simulink model "Clutchless_P2_Parallel_ETE"  (R2017b)
settings: Solver=FixedStepAuto  StartTime=0.0  StopTime=length(Speed)  FixedStep=0.01  MaxStep=0.01  RelTol=1e-3  EnableMultiTasking=on
PostLoadFcn:
  | , if any(exist('dsrtsu_mdlpostloadfcn', 'file') == [2, 3, 6]), try dsrtsu_mdlpostloadfcn('Execute', bdroot); catch fprintf('Error in PostLoadFcn (dsrtsu_mdlpostloadfcn) for model "%s":\n %s\n', bdroot, lasterr); end, end,
undefined symbols (not defined in the file): ABSEnable, Actuators, air, APP1_OOR, APP2_OOR, APP_Mismatch, Brk_Flt, cal, ClutchEngag, Clutchless_HSC_ETE, CS_On_Control, Driver, eng, Engine, EngOverTemp, ENGTRQ_MSMCH_Degraded_CP, ENGTRQ_MSMCH_ErrCritical_CP, ENGTRQ_MSMCH_LimpHome_CP, EngTrqMismatch, env, ess, ESSOverTemp, gb, KeyPos_Flt, KeyPosition, lib_Actuators, lib_Clutchless_HSC_ETE, lib_Driver, lib_EMachine_2017a, lib_Sensors_2017a, LossCAN, Machine, max_vehicle_rad_air_flow, MCUOverTemp, mot, MotDirMismatch, MotOverTemp, MotTrqMismatch, mph2ms, PRNDL_Flt, RegenBrkDisable, RegenFault, Sensors, ShiftLeverPosition, Speed, SW_CS_ON, SW_Engine_ON, t_amb, time, tloop
libraries: simulink x97, Pneumatic_lib x11, nesl_utility x9, EC2_libraries x7, powerlib_meascontrol x2, CalculationGallon x1, lib_Chassis x1, lib_DCDC x1, lib_Differential x1, lib_HVESS x1, fl_lib x1, lib_OBC x1
(part 3 of 9)

== system Clutchless_P2_Parallel_ETE/Camaro Plant Model/ICE Simple1/Engine Plant Modified/ECU Sensors ==
  In1 : Inport
  In2 : Inport  Port=2
  In3 : Inport  Port=3
  In4 : Inport  Port=4
  In5 : Inport  Port=5
  In6 : Inport  Port=6
  In7 : Inport  Port=7
  In8 : Inport  Port=8
  In9 : Inport  Port=9
  In10 : Inport  Port=10
  Bus Creator : BusCreator  Inputs=10
  Memory : Memory
  Out1 : Outport
  wires:
  In9/1 -> Bus Creator/9  "NOx_g/s"
  In1/1 -> Bus Creator/1  "EngActStdyStTorq_Nm"
  In2/1 -> Bus Creator/2  "EngSpd_RPM"
  In3/1 -> Bus Creator/3  "EngFuelFlow_g/s"
  In4/1 -> Bus Creator/4  "FuelLevelPct"
  In5/1 -> Bus Creator/5  "PE_0_1"
  In6/1 -> Bus Creator/6  "HC_g/s"
  In7/1 -> Bus Creator/7  "CO_g/s"
  Bus Creator/1 -> Memory/1
  In8/1 -> Bus Creator/8  "CO2_g/s"
  In10/1 -> Bus Creator/10  "Eng_Temp"
  Memory/1 -> Out1/1

== system Clutchless_P2_Parallel_ETE/Camaro Plant Model/ICE Simple1/Engine Plant Modified/Fuel Supply ==
  0 to 100 : Saturate
  Fuel Pump Disable : Constant  Value=0
  Fuel Volumn : Constant  Value=Engine.Fuel.Initial_Volumn
  Integrator : Integrator  LimitOutput=on  UpperSaturationLimit=Engine.FuelTank.Volume  LowerSaturationLimit=0
  L to % : Gain  Gain=100/Engine.FuelTank.Volume
  Sum : Sum  Inputs=+-
  Switch : Switch  Threshold=1
  g to L : Gain  Gain=1/Engine.Fuel.Density/1000
  Available Fuel : Outport
  tag scope: FuelLevelPct=global
  wires:
  0 to 100/1 -> [FuelLevelPct]
  L to %/1 -> 0 to 100/1
  Fuel Pump Disable/1 -> Switch/3
  g to L/1 -> Switch/1
  Integrator/1 -> g to L/1
  [AdvFuelFlowEst] -> Integrator/1
  [FuelPumpEnable] -> Switch/2
  Sum/1 -> L to %/1, Available Fuel/1
  Switch/1 -> Sum/2
  Fuel Volumn/1 -> Sum/1

== system Clutchless_P2_Parallel_ETE/Camaro Plant Model/ICE Simple1/Engine Plant Modified/Radiator ==
  note: Calculation of max air flow:
      |
      | The air flow reach the max in the scenario that only fan rejects all the heat coolant brings in
      |
      | The regular max CFM of a vehicle radiator fan is about 2000
      |
      | CFM=1.76* Q/delta T_air
      |
      | Where Q is the max amount of heat from coolant, assume that the max temperature drop of coolant
      | through radiator is 10 deg C
      |
      | Q= Mc_coolant* Cp_coolant* delta T_coolant=3500*0.26*10=9100w
      |
      | delta T_air=1.76*Q/CFM=1.76*9100/2000=8 degC
      |
      | Max Mc_air=Q/(Cp_air*delta T_air)=9100/(1006*8)=1.13 kg/s
  EngCltTmp : Inport
  Fans : Inport  Port=2
  " " : Product  Inputs=**
  " " : Gain  Gain=0.05
  Ambient Temp : Constant  Value=env.init.T_ambiant
  Compare To Zero : simulink/Logic and Bit Operations/Compare To Zero  relop===  OutDataTypeStr=uint8
  Constant : Constant
  Cp of Air : Constant  Value=air.init.specific_heat
  Cp of Air1 : Constant  Value=air.init.specific_heat
  Data Type Conversion1 : DataTypeConversion
  Divide by Zero Fix : Subsystem
  "Eng Mc=Q/(Cp*delta T) " : Product  Inputs=*/
  Q=Mc_air*Cp_air*delta T : Product  Inputs=***
  Saturation : Saturate  UpperLimit=max_vehicle_rad_air_flow  LowerLimit=-1
  Sum3 : Sum  Inputs=|-+
  Sum4 : Sum
  Sum5 : Sum  Inputs=|+-
  Switch : Switch  Threshold=1
  Terminator : Terminator
  vehspdflow : Gain  Gain=0.01
  tag scope: AirFlowRequest=global, Heat_Reject_Eng=global
  wires:
  Data Type Conversion1/1 -> " "/1
  Cp of Air1/1 -> Q=Mc_air*Cp_air*delta T/3
  Switch/1 -> Q=Mc_air*Cp_air*delta T/2  "eng act air flow in kg/s"
  Q=Mc_air*Cp_air*delta T/1 -> " "/2  "J/s"
  " "/1 -> [Heat_Reject_Eng]  "J"
  Saturation/1 -> Sum3/1  "Actual air flow"
  Sum3/1 -> Compare To Zero/1
  Compare To Zero/1 -> Switch/2  "request meet"
  Cp of Air/1 -> "Eng Mc=Q/(Cp*delta T) "/2  "Cp J/kg*C"
  Ambient Temp/1 -> Sum5/2  "25 deg C"
  Sum5/1 -> Divide by Zero Fix/2(Divide), Q=Mc_air*Cp_air*delta T/1  "Delta T = Tcoolant - Tambient"
  EngCltTmp/1 -> Sum5/1  "EngCltTmp in deg C"
  "Eng Mc=Q/(Cp*delta T) "/1 -> Switch/1, Sum3/2, [AirFlowRequest]  "Eng requested air flow in Kg/s"
  Sum4/1 -> Switch/3, Saturation/1  "Air Flow Recieved"
  Fans/1 -> Data Type Conversion1/1
  [VehSpdAvgDrvn_Eng] -> vehspdflow/1
  vehspdflow/1 -> Sum4/2
  [Heat_Transfer_Eng] -> Divide by Zero Fix/1(Multiply)  "heat generation in w"
  Divide by Zero Fix/1(Output) -> "Eng Mc=Q/(Cp*delta T) "/1
  " "/1 -> Sum4/1
  Constant/1 -> " "/1
  [AirFlowRequest] -> Terminator/1

== system Clutchless_P2_Parallel_ETE/Camaro Plant Model/ICE Simple1/Engine Plant Modified/Subsystem ==
  EngFuelFlow_g/s : Inport
  Eng_Temp : Inport  Port=2
  Rate Transition1 : RateTransition  OutPortSampleTime=1
  Rate Transition7 : RateTransition  OutPortSampleTime=1
  To Workspace2 : ToWorkspace  VariableName=EngCltTmp  SampleTime=-1
  To Workspace3 : ToWorkspace  VariableName=InstFuelConsmpRate  SampleTime=-1
  g/s 2 l/hr : Gain  Gain=0.001/0.7871*3600
  wires:
  EngFuelFlow_g/s/1 -> g/s 2 l/hr/1
  Eng_Temp/1 -> Rate Transition1/1
  Rate Transition1/1 -> To Workspace2/1
  g/s 2 l/hr/1 -> Rate Transition7/1
  Rate Transition7/1 -> To Workspace3/1

== system Clutchless_P2_Parallel_ETE/Camaro Plant Model/ICE Simple1/Inputs/Analog ==
  Out1 : Outport
  wires:
  [Analog] -> Out1/1

== system Clutchless_P2_Parallel_ETE/Camaro Plant Model/ICE Simple1/Inputs/CAN_from_HCU ==
  Bus Creator : BusCreator  Inputs=2
  Out1 : Outport
  wires:
  [HCU_to_EBCAN] -> Bus Creator/1
  [HCU_to_VEH_CAN] -> Bus Creator/2
  Bus Creator/1 -> Out1/1

== system Clutchless_P2_Parallel_ETE/Camaro Plant Model/ICE Simple1/Soft ECM/ECM_RollingAliveCnt ==
  Constant : Constant
  Constant1 : Constant  Value=0
  Rolling Alive Counter : Stateflow chart  TreatAsAtomicUnit=on
  Switch : Switch  Criteria=u2 > Threshold
  Out1 : Outport
  tag scope: ECM_CAN_fault=global
  wires:
  [ECM_CAN_fault] -> Switch/2
  Constant/1 -> Switch/1
  Rolling Alive Counter/1(RollingAliveCnt) -> Switch/3
  Switch/1 -> Out1/1  "ECM_RollingAliveCnt"
  Constant1/1 -> [ECM_CAN_fault]

== system Clutchless_P2_Parallel_ETE/Camaro Plant Model/ICE Simple1/Soft ECM/Fuel Consumption ==
  note: Total Fuel Consumed
  Fuel Consumption : Inport
  " " : Constant  Value=3600
  " tloop" : Constant  Value=0.01
  1/fuel density : Gain  Gain=1/Engine.Fuel.Density
  Add : Sum  Inputs=|++
  Add1 : Sum  Inputs=|++
  Constant3 : Constant  Value=Engine.Fuel.Lower_Heating_Value/1000
  Divide : Product  Inputs=*/
  Divide by Zero Fix : Subsystem
  Divide by Zero Fix1 : Subsystem
  Gain1 : Gain  Gain=0.001
  Memory : Memory
  Memory1 : Memory
  Product : Product  RndMeth=Zero
  Product1 : Product  RndMeth=Zero
  Product3 : Product  RndMeth=Zero
  Scope : Scope
  To Workspace1 : ToWorkspace  VariableName=eng_fuel_consump_mpl  SampleTime=-1
      settings: Decimation=WORKSPACE_DECIMATION
  To Workspace5 : ToWorkspace  VariableName=eng_wh_per_mile_hist  SampleTime=-1
      settings: Decimation=WORKSPACE_DECIMATION
  fuel consumption : Outport
  wires:
  Divide by Zero Fix1/1(Output) -> To Workspace5/1
  Divide/1 -> Add1/1  "Wh"
  Memory1/1 -> Add1/2
  Add1/1 -> Divide by Zero Fix1/2(Multiply), Memory1/1  "cumulative"
  Product/1 -> Product3/2  "W"
  Constant3/1 -> Product/2
  Divide by Zero Fix/1(Output) -> fuel consumption/1, To Workspace1/1, Scope/1
  [veh_dist_miles] -> Divide by Zero Fix1/1(Divide), Divide by Zero Fix/2(Multiply)  "miles"
  Product1/1 -> Add/1  "liter"
  1/fuel density/1 -> Product1/1  "liter/sec"
  Fuel Consumption/1 -> Product/1, Gain1/1  "g/s"
  Memory/1 -> Add/2
  Add/1 -> Divide by Zero Fix/1(Divide), Memory/1  "cumulative_liter"
  " tloop"/1 -> Product3/1, Product1/2
  Product3/1 -> Divide/1
  " "/1 -> Divide/2
  Gain1/1 -> 1/fuel density/1

== system Clutchless_P2_Parallel_ETE/Camaro Plant Model/ICE Simple1/Soft ECM/Logic/APP2TP ==
  APP : Inport
  EngSpd : Inport  Port=2
  f : TriggerPort  TriggerType=function-call  VariantControl=Variant
      settings: CopyFcn=Stateflow.SLINSF.SimulinkMan.removeBlockPreDeleteFcn  PreDeleteFcn=Stateflow.SLINSF.SimulinkMan.unsafePredeleteFcn
  Based on APP to TP test data from 2013 Malibu1 : Lookup_n-D  NumberOfTableDimensions=1  BreakpointsForDimension1=[0,1,2,3,4,5,6,7,8,9,10,11,12,13,14,15,16,17,18,19,20,21,22,23,24,25,26,27,28,29,30,31,32,33,34,35,36,37,38,39,40,41,42,43,44,45,46,48,51,55,60,66,100]  Table=[0,6.3,12.7686537241448,12.6326703204763,12.8888951657611,13.4307541011932,14.1739282202018,15.0532596030224,16.0198646102832,17.0384547356068,18.0848650172271,19.1437900086214,20.206727308158,21.2701286477589,22.3337585405773,23.3992604876916,24.4689307438132,25.5446996420107,26.6273204774486,27.7157659501418,28.8068321667249,29.8949502012373,30.9722052149229,32.0285631350456,33.0523048927199,34.0306682197568,34.9506970045247,35.8002982068255,36.5695063317874,37.2519554627699,37.846558853288,38.359396077948,38.8058077424007,39.2126977523099,39.6210431413345,40.0886114581279,40.6928857123509,41.5341968797017,42.7390639659588,44.4637416300428,46.8979753660875,50.2689642445339,54.8455312122302,60.9425009515619,68.9252852985734,79.2146762201353,81.9427,84.6943,87.2166,89.5096,91.3439,92.6051,100]  ExtrapMethod=Clip  UseLastTableValue=on  InternalRulePriority=Speed  RndMeth=Simplest  InputSameDT=on
  Based on APP to TP test data from 2013 Malibu2 : Lookup_n-D  Commented=on  NumberOfTableDimensions=1  BreakpointsForDimension1=[0,1,2,3,4,5,6,7,8,9,10,11,12,13,14,15,16,17,18,19,20,21,22,23,24,25,26,27,28,29,30,31,32,33,34,35,36,37,38,39,40,41,42,43,44,45,46,48,51,55,60,66,100]  Table=[0,7,12.5,16,16.5,17,18,19,21,23,25,28,29,30,32,35,37,39,41,44,47,48,48.6,49,50,51.5,52,53,53.25,53.5,55,56.75,57,58,60,64,68,72,73,74,75,76,77,77.5,78,80,82,85,87,89.5,91.5,93,100]  ExtrapMethod=Clip  UseLastTableValue=on  InternalRulePriority=Speed  RndMeth=Simplest  InputSameDT=on
  Display : Display
  Product : Product
  RPM Derating : Lookup_n-D  NumberOfTableDimensions=1  BreakpointsForDimension1=[0 1000 2000 3000 4000 5000 6000 7000]  Table=[1 1 1 1 1 1 1 0]  ExtrapMethod=Clip  UseLastTableValue=on  InternalRulePriority=Speed  RndMeth=Simplest  InputSameDT=on
  Saturation : Saturate  UpperLimit=100  LowerLimit=0
  TP : Outport
  wires:
  Product/1 -> TP/1
  EngSpd/1 -> RPM Derating/1
  RPM Derating/1 -> Product/2  "2"
  APP/1 -> Based on APP to TP test data from 2013 Malibu1/1, Display/1  "3"
  Based on APP to TP test data from 2013 Malibu1/1 -> Saturation/1  "1"
  Saturation/1 -> Product/1

== system Clutchless_P2_Parallel_ETE/Camaro Plant Model/Scopes/AxlTrq_to_EngTrq2/Ratio Filter ==
  Ratio : Inport
  Abs : Abs
  Compare To Zero : simulink/Logic and Bit Operations/Compare To Zero  relop===  OutDataTypeStr=boolean
  Constant : Constant  Value=cal.Time.TrnsOvrllEstTrqRatioSwitch
  Mature_Delay : EC2_libraries/Mature_Delay
      settings: SourceProductName=The database C:\Users\vrajm\AppData\Roaming\MathWorks\MATLAB\R2017b\slblocks_master.db is locked, or a table in the database is locked. (database is locked)
  Memory1 : Memory  InitialCondition=1
  Switch1 : Switch  Threshold=1
  Switch2 : Switch  Threshold=1
  Filtered_Ratio : Outport
  wires:
  Ratio/1 -> Compare To Zero/1, Abs/1
  Compare To Zero/1 -> Mature_Delay/1, Switch2/2
  Abs/1 -> Switch1/1, Switch2/3
  Switch1/1 -> Switch2/1
  Constant/1 -> Mature_Delay/2
  Mature_Delay/1 -> Switch1/2
  Memory1/1 -> Switch1/3
  Switch2/1 -> Filtered_Ratio/1, Memory1/1  "gear_ratio"

== system Clutchless_P2_Parallel_ETE/Camaro Plant Model/Scopes/AxlTrq_to_MtrTrq2/Ratio Filter ==
  Ratio : Inport
  Abs : Abs
  Compare To Zero : simulink/Logic and Bit Operations/Compare To Zero  relop===  OutDataTypeStr=boolean
  Constant : Constant  Value=cal.Time.TrnsOvrllEstTrqRatioSwitch
  Mature_Delay : EC2_libraries/Mature_Delay
      settings: SourceProductName=The database C:\Users\vrajm\AppData\Roaming\MathWorks\MATLAB\R2017b\slblocks_master.db is locked, or a table in the database is locked. (database is locked)
  Memory1 : Memory  InitialCondition=1
  Switch1 : Switch  Threshold=1
  Switch2 : Switch  Threshold=1
  Filtered_Ratio : Outport
  wires:
  Ratio/1 -> Compare To Zero/1, Abs/1
  Compare To Zero/1 -> Mature_Delay/1, Switch2/2
  Abs/1 -> Switch1/1, Switch2/3
  Switch1/1 -> Switch2/1
  Constant/1 -> Mature_Delay/2
  Mature_Delay/1 -> Switch1/2
  Memory1/1 -> Switch1/3
  Switch2/1 -> Filtered_Ratio/1, Memory1/1  "gear_ratio"

== system Clutchless_P2_Parallel_ETE/Clutchless_HSC_ETE/HSC/Camaro Fault Detection/Component Diagnostic ==
  note: Component Status Setting Rule
      | xxx_CompStatus could be 0, 1, 2 or 3
      | 0: component needs to be offline
      | 1: component needs torque plant to deliver creep torque
      | 2: component needs torque plant to limit maximum torque delivery
      | 3: component needs torque plant to operate normally
  note: Component Diagnostics
  SignalDiag : Inport
  Bus Creator : BusCreator  Inputs=6
  Driver Input Diagnostic : Subsystem
  ESS Component Diagnostic : Subsystem
  Engine Component Diagnostic : Subsystem
  Override Driver Status : Subsystem
  Override ESS Status : Subsystem
  Override Engine Status : Subsystem
  Override TCM Status : Subsystem
  Transmission Component Diagnostic : Subsystem
  CompDiag : Outport
  wires:
  SignalDiag/1 -> Engine Component Diagnostic/1(In1), Transmission Component Diagnostic/1(In1), Bus Creator/6, ESS Component Diagnostic/1(In1), Driver Input Diagnostic/1(In1)  "RawSig"
  Bus Creator/1 -> CompDiag/1
  Driver Input Diagnostic/1(Out1) -> Override Driver Status/1(In1)  "Diver_CompDiag"
  ESS Component Diagnostic/1(Out1) -> Override ESS Status/1(In1)  "ESS_CompDiag"
  Engine Component Diagnostic/1(Out1) -> Override Engine Status/1(In1)  "ECM_CompDiag"
  Transmission Component Diagnostic/1(Out1) -> Override TCM Status/1(In1)  "TCM_CompDiag"
  Override ESS Status/1(Out1) -> Bus Creator/2  "BMS_Status"
  Override Engine Status/1(Out1) -> Bus Creator/3  "ECM_Status"
  Override TCM Status/1(Out1) -> Bus Creator/5  "TCM_Status"
  Override Driver Status/1(Out1) -> Bus Creator/1  "Driver_Input_Status"
  Engine Component Diagnostic/2(Out2) -> Bus Creator/4  "EngTrqMismchType"

== system Clutchless_P2_Parallel_ETE/Clutchless_HSC_ETE/HSC/Camaro Fault Detection/Input Conversions ==
  note: Input Conversions and Override Switches
  note: These subsystems convert variable types to match those used in the
      | supervisor. In addition, override switches installed on each signal can
      | be used to manually override and signal for testing purposes
  RawSig : Inport
  BMS_Conversions : Subsystem
  Bus Creator : BusCreator  Inputs=5
  DriverInput_Conversions : Subsystem
  ECM_Conversions : Subsystem
  TCM_Conversions : Subsystem
  VehSig : Outport
  wires:
  DriverInput_Conversions/1(Out1) -> Bus Creator/1
  Bus Creator/1 -> VehSig/1  "InputConvAndOvrd"
  BMS_Conversions/1(Out1) -> Bus Creator/2
  RawSig/1 -> DriverInput_Conversions/1(In1), Bus Creator/5, TCM_Conversions/1(In1), ECM_Conversions/1(In1), BMS_Conversions/1(In1)  "RawSig"
  ECM_Conversions/1(Out1) -> Bus Creator/3
  TCM_Conversions/1(Out1) -> Bus Creator/4

== system Clutchless_P2_Parallel_ETE/Clutchless_HSC_ETE/HSC/Camaro Fault Detection/Signal Diagnostic ==
  note: These subsystems evaluate each signal for proper value range and other checks
  note: Signal Diagnostics
  VehSig : Inport
  Bus Creator : BusCreator  Inputs=5
  Driver Signal Diagnostic : Subsystem
  ESS Signal Diagnostic : Subsystem
  Engine Signal Diagnostic : Subsystem
  Subsystem1 : Subsystem
      mask Display: fprintf('Signal Naming Rule')
  Transmission Signal Diagnostic : Subsystem
  SignalDiag : Outport
  wires:
  VehSig/1 -> ESS Signal Diagnostic/1(Sensors1), Driver Signal Diagnostic/1(Sensors1), Engine Signal Diagnostic/1(Sensors1), Bus Creator/5, Transmission Signal Diagnostic/1(Sensors1)
  Driver Signal Diagnostic/1(Driver_SigDiag) -> Bus Creator/1  "Driver_SigDiag"
  ESS Signal Diagnostic/1(ESS_SigDiag) -> Bus Creator/2  "ESS_SigDiag"
  Engine Signal Diagnostic/1(Engine_SigDiag) -> Bus Creator/3  "Engine_SigDiag"
  Transmission Signal Diagnostic/1(Out2) -> Bus Creator/4  "Transmission_SigDiag"
  Bus Creator/1 -> SignalDiag/1  "SignalDiag"

== system Clutchless_P2_Parallel_ETE/Clutchless_HSC_ETE/HSC/Driver_Requests/APP_BPP to DrvIntndAxlTrq2 ==
  note: $Author: fy6949 $
      | $Rev: 577 $
      | $Date: 2017-1-19 08:53:15 -0500  $
  note: Note:Driver requested Axle Torque Calculation
  Sensors : Inport
  Diag : Inport  Port=2
  Controls : Inport  Port=3
  Bus Selector : BusSelector  OutputSignals=from_Analog.Driver_APP1,from_CAN.fromVEH_CAN.from_BCM.BrkPdlPos,from_CAN.fromEBCAN.from_ECM.VehSpdAvgDrvn,from_CAN.fromVEH_CAN.from_TCM.TrnGrRat,from_CAN.fromHV_CAN.from_MCU.INV_VCU_01.INV_Speed
  Bus Selector1 : BusSelector  OutputSignals=CompSig.RawSig.Driver_SigDiag.Drv_APP_Agree
  Bus Selector2 : BusSelector  OutputSignals=mode
  Post Driver Intnded Axle Torque : Subsystem
  Terminator : Terminator
  Terminator1 : Terminator
  IntndAxlTrq : Outport
  wires:
  Bus Selector2/1 -> Post Driver Intnded Axle Torque/5(Mode)  "<mode>"
  Bus Selector1/1 -> Terminator1/1  "<Drv_APP_Agree>"
  Diag/1 -> Bus Selector1/1
  Post Driver Intnded Axle Torque/2(BrkIntndAxlTrq) -> Terminator/1
  Bus Selector/1 -> Post Driver Intnded Axle Torque/1(APP)  "<Driver_APP1>"
  Bus Selector/4 -> Post Driver Intnded Axle Torque/4(TransGearRatio)  "<TrnGrRat>"
  Bus Selector/5 -> Post Driver Intnded Axle Torque/6(Motor_Speed)  "<INV_Speed>"
  Bus Selector/3 -> Post Driver Intnded Axle Torque/3(VehicleSpeed)  "<VehSpdAvgDrvn>"
  Bus Selector/2 -> Post Driver Intnded Axle Torque/2(BPP)  "<BrkPdlPos>"
  Post Driver Intnded Axle Torque/1(IntndAxlTrq) -> IntndAxlTrq/1
  Controls/1 -> Bus Selector2/1
  Sensors/1 -> Bus Selector/1

== system Clutchless_P2_Parallel_ETE/Clutchless_HSC_ETE/HSC/Powertrain Manager/HV Manager1 ==
  Sensors : Inport
  Controls : Inport  Port=2
  Axiomatic_Output_Manager : Subsystem
  BMS_Manager : Subsystem
  Bus Creator1 : BusCreator  Inputs=4
  DCDC Manager : Subsystem
  Inverter Manager : Subsystem
  OBC_Manager : Subsystem
  BMS_CAN : Outport
  HV_BUS_Status : Outport  Port=2
  OBC_CAN : Outport  Port=3
  OBC_Digital : Outport  Port=4
  BMS_Digital : Outport  Port=5
  Axiomatic_CAN : Outport  Port=6
  tag scope: MCU_CAN=global
  wires:
  [MCU_Status] -> BMS_Manager/3(In1)
  DCDC Manager/1(Out1) -> Bus Creator1/4
  Inverter Manager/3(MCU_Relay) -> Bus Creator1/3  "MCU_Relay"
  Axiomatic_Output_Manager/1(Axiomatic_CAN) -> Axiomatic_CAN/1
  BMS_Manager/3(BMS Digital) -> BMS_Digital/1
  BMS_Manager/1(BMS CAN) -> BMS_CAN/1
  Controls/1 -> Inverter Manager/3(Control), DCDC Manager/3(In2), DCDC Manager/2(In1), BMS_Manager/2(Controls)
  OBC_Manager/2(OBC_Digital) -> OBC_Digital/1
  OBC_Manager/1(OBC CAN) -> OBC_CAN/1
  [HV_BUS_Status] -> OBC_Manager/1(HV_Status)
  BMS_Manager/2(HV_BUS_Status) -> HV_BUS_Status/1, [HV_BUS_Status]  "HV_BUS_Status"
  [HV_BUS_Status] -> Axiomatic_Output_Manager/2(HV_Bus_Status)
  [HV_BUS_Status] -> Inverter Manager/1(HV_Bus_Status)  "HV_BUS_Status"
  Sensors/1 -> Inverter Manager/2(Sensors), OBC_Manager/2(Sensors), Axiomatic_Output_Manager/1(Sensors), DCDC Manager/1(BMSInput), BMS_Manager/1(Sensors)
  Inverter Manager/1(MCU_Status) -> Bus Creator1/1, [MCU_Status]  "MCU_Status"
  Inverter Manager/2(MCU_CAN) -> Bus Creator1/2  "MCU_CAN"
  Bus Creator1/1 -> [MCU_CAN]

== system Clutchless_P2_Parallel_ETE/Clutchless_HSC_ETE/HSC/Powertrain Manager/Output Conversion ==
  In1 : Inport
  In2 : Inport  Port=2
  In3 : Inport  Port=3
  In4 : Inport  Port=4
  In5 : Inport  Port=5
  In8 : Inport  Port=6
  In9 : Inport  Port=7
  In10 : Inport  Port=8
  In11 : Inport  Port=9
  Bus Creator : BusCreator  Inputs=14
  Bus Creator1 : BusCreator  Inputs=9
  Bus Selector2 : BusSelector  OutputSignals=powerMode,EnablePrplsn,ClutchEngage,EngAppReq,EngOnReq,MtrTrqCmd,EnableInverter,EngTrqCmd,HV_req,SysPwrMd_0_3,TransShftLvrPos,VehSpdAvgDrvn_kph,AccPos_Perc,SportsModeEnable
  Data Type Conversion{,2..3,5..13} (12 alike) : DataTypeConversion
  Memory : Memory
  Out1 : Outport
  wires:
  Bus Selector2/14 -> Bus Creator/14  "<SportsModeEnable>"
  In11/1 -> Bus Creator1/9
  In4/1 -> Bus Selector2/1
  Bus Selector2/1 -> Memory/1  "<powerMode>"
  Bus Selector2/2 -> Data Type Conversion2/1  "<EnablePrplsn>"
  Bus Selector2/3 -> Data Type Conversion3/1  "<ClutchEngage>"
  Bus Selector2/5 -> Data Type Conversion5/1  "<EngOnReq>"
  Bus Selector2/6 -> Data Type Conversion6/1  "<MtrTrqCmd>"
  Bus Selector2/7 -> Data Type Conversion7/1  "<EnableInverter>"
  Bus Selector2/8 -> Data Type Conversion8/1  "<EngTrqCmd>"
  Bus Selector2/9 -> Data Type Conversion9/1  "<HV_req>"
  Bus Selector2/10 -> Data Type Conversion10/1  "<SysPwrMd_0_3>"
  Data Type Conversion2/1 -> Bus Creator/2  "EnablePrplsn"
  Data Type Conversion3/1 -> Bus Creator/3  "ClutchEngage"
  Bus Selector2/4 -> Bus Creator/4  "<EngAppReq>"
  Data Type Conversion6/1 -> Bus Creator/6  "Torque_Command"
  Data Type Conversion7/1 -> Bus Creator/7  "Inverter_Enable"
  Data Type Conversion8/1 -> Bus Creator/8  "EngTrqCmd"
  Data Type Conversion9/1 -> Bus Creator/9  "HV_req"
  Data Type Conversion10/1 -> Bus Creator/10  "SysPwrMd"
  Data Type Conversion/1 -> Bus Creator/1  "powerMode"
  Data Type Conversion5/1 -> Bus Creator/5  "EngOnReq"
  Bus Creator1/1 -> Out1/1
  In1/1 -> Bus Creator1/1
  In2/1 -> Bus Creator1/2
  In3/1 -> Bus Creator1/3
  Bus Creator/1 -> Bus Creator1/4  "Controls"
  In5/1 -> Bus Creator1/5
  Bus Selector2/11 -> Data Type Conversion11/1  "<TransShftLvrPos>"
  Data Type Conversion11/1 -> Bus Creator/11  "ShftLvrPos"
  Bus Selector2/12 -> Data Type Conversion12/1  "<VehSpdAvgDrvn_kph>"
  Data Type Conversion12/1 -> Bus Creator/12  "VehSpdAvgDrvn_kph"
  Bus Selector2/13 -> Data Type Conversion13/1  "<AccPos_Perc>"
  Data Type Conversion13/1 -> Bus Creator/13  "AccPos_Perc"
  Memory/1 -> Data Type Conversion/1
  In8/1 -> Bus Creator1/6
  In9/1 -> Bus Creator1/7
  In10/1 -> Bus Creator1/8

== system Clutchless_P2_Parallel_ETE/Clutchless_HSC_ETE/HSC/Powertrain Manager/Thermal Manager ==
  In2 : Inport
  Bus Creator : BusCreator  Inputs=3
  Bus Creator1 : BusCreator  Inputs=4
  Bus Creator2 : BusCreator  Inputs=4
  Bus Creator3 : BusCreator  Inputs=3
  Bus Creator4 : BusCreator  Inputs=1
  Bus Selector : BusSelector  OutputSignals=from_CAN.fromEBCAN.from_ECM.EngCltTmp,from_CAN.fromHV_CAN.from_BMSHybrid.BMS_Temperatur,from_CAN.fromHV_CAN.from_MCU.INV_VCU_04.INV_InverterTemperature,from_CAN.fromHV_CAN.from_MCU.INV_VCU_04.INV_ElectricMachineTemperature,from_CAN.fromEBCAN.from_ECM.EngRunAtv,from_CAN.fromHV_CAN.from_BMSHybrid.BMS_HYB_02.BMS_IstModus,from_CAN.fromVEH_CAN.from_BCM.SysPwrMd,from_CAN.fromEBCAN.from_ECM.VehSpdAvgDrvn
  Bus Selector3 : BusSelector  OutputSignals=from_CAN.fromHV_CAN.from_BMSHybrid.BMS_HYB_02.BMS_Fehler_Pilot
  Compare To Constant1 : simulink/Logic and Bit Operations/Compare To Constant  relop=>  const=0  OutDataTypeStr=boolean
  Cooling Fan Manger : Subsystem
  Data Type Conversion : DataTypeConversion  OutDataTypeStr=double
  ESS Pump Manger : Subsystem
  MotInv Pump Manger : Subsystem
  Out1 : Outport
  wires:
  Compare To Constant1/1 -> Data Type Conversion/1
  Data Type Conversion/1 -> Bus Creator4/1  "FuelPump_Disable"
  Bus Creator4/1 -> Bus Creator1/4  "Pump_Commands"
  Bus Selector3/1 -> Compare To Constant1/1  "<BMS_Fehler_Pilot>"
  In2/1 -> Bus Selector/1, Bus Selector3/1
  Bus Creator3/1 -> Bus Creator/2  "Component_State"
  Bus Creator2/1 -> Bus Creator/1  "Temp_Signals"
  MotInv Pump Manger/1(MotInvpump_control) -> Bus Creator1/3  "MotMCU_Pump_Control"
  ESS Pump Manger/1(ESS_Thermal_Control) -> Bus Creator1/2  "ESS_Pump_Control"
  Bus Creator/1 -> MotInv Pump Manger/1(MotInv_temp), ESS Pump Manger/1(ESS_temp), Cooling Fan Manger/1(Temp)
  Cooling Fan Manger/1(Fan_control) -> Bus Creator1/1  "Fan_Control"
  Bus Creator1/1 -> Out1/1  "Thermal_Control"
  Bus Selector/1 -> Bus Creator2/1  "<EngCltTmp>"
  Bus Selector/2 -> Bus Creator2/2  "<BMS_Temperatur>"
  Bus Selector/3 -> Bus Creator2/3  "<INV_InverterTemperature>"
  Bus Selector/4 -> Bus Creator2/4  "<INV_ElectricMachineTemperature>"
  Bus Selector/5 -> Bus Creator3/1  "<EngRunAtv>"
  Bus Selector/6 -> Bus Creator3/2  "<BMS_IstModus>"
  Bus Selector/7 -> Bus Creator3/3  "<SysPwrMd>"
  Bus Selector/8 -> Bus Creator/3  "<VehSpdAvgDrvn>"

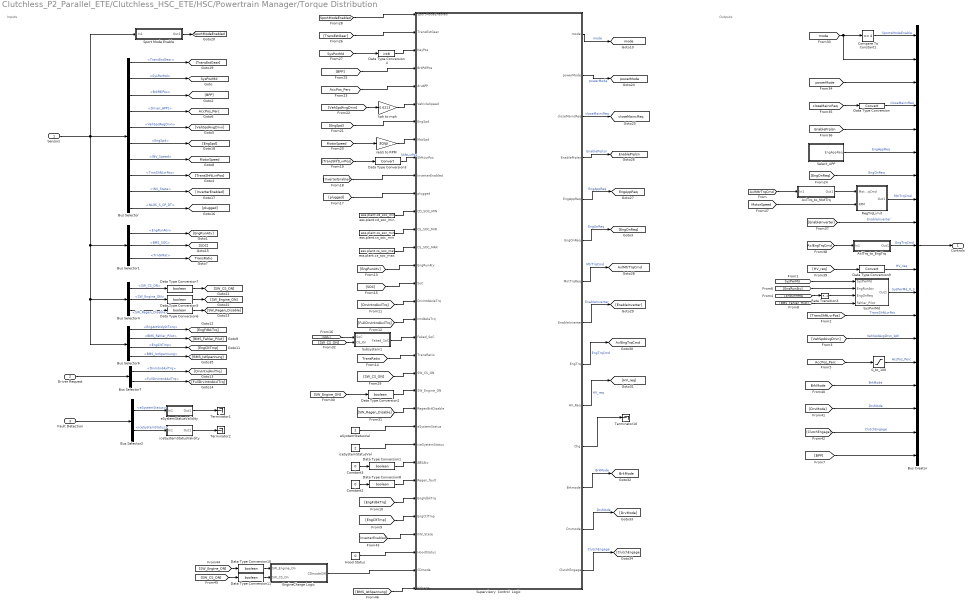
== system Clutchless_P2_Parallel_ETE/Clutchless_HSC_ETE/HSC/Powertrain Manager/Torque Distribution ==
  note: Inputs
  note: Outputs
  Sensors : Inport
  Driver Request : Inport  Port=2
  Fault Detection : Inport  Port=3
  0_to_100 : Saturate  UpperLimit=100  LowerLimit=0
  AxlTrq_to_EngTrq : Subsystem
  AxlTrq_to_MotTrq : Subsystem
  Bus Creator : BusCreator  Inputs=19
  Bus Selector : BusSelector  OutputSignals=from_CAN.fromVEH_CAN.from_TCM.TransEstGear,from_CAN.fromVEH_CAN.from_BCM.SysPwrMd,from_CAN.fromVEH_CAN.from_BCM.BrkPdlPos,from_Analog.Driver_APP1,from_CAN.fromEBCAN.from_ECM.VehSpdAvgDrvn,from_CAN.fromEBCAN.from_ECM.EngSpd,from_CAN.fromHV_CAN.from_MCU.INV_VCU_01.INV_Speed,from_CAN.fromVEH_CAN.from_TCM.TrnsShftLvrPos,from_CAN.fromHV_CAN.from_MCU.INV_VCU_01.INV_State,from_CAN.fromHV_CAN.from_OBC.NLG5_ST.NLG5_S_CP_DT
  Bus Selector1 : BusSelector  OutputSignals=from_CAN.fromEBCAN.from_ECM.EngRunAtv,from_CAN.fromHV_CAN.from_BMSHybrid.BMS_SOC,from_CAN.fromVEH_CAN.from_TCM.TrnGrRat
  Bus Selector2 : BusSelector  OutputSignals=eSystemDiagOut.eSystemStatus,iceSystemDiagOut.iceSystemStatus
  Bus Selector4 : BusSelector  OutputSignals=from_Digital.SW_CS_ON,from_Digital.SW_Engine_ON,from_Digital.SW_Regen_Disable
  Bus Selector6 : BusSelector  OutputSignals=from_CAN.fromEBCAN.from_ECM.EngActStdyStTorq,from_CAN.fromHV_CAN.from_BMSHybrid.BMS_HYB_02.BMS_Fehler_Pilot,from_CAN.fromEBCAN.from_ECM.EngCltTmp,from_CAN.fromHV_CAN.from_BMSHybrid.BMS_HYB_02.BMS_IstSpannung
  Bus Selector7 : BusSelector  OutputSignals=DrvIntndAxlTrq,FullDrvIntndAxlTrq
  Compare To Constant1 : simulink/Logic and Bit Operations/Compare To Constant  relop===  const=4  OutDataTypeStr=boolean
  Constant2 : Constant  Value=0
  Constant3 : Constant  Value=0
  Data Type Conversion : DataTypeConversion
  Data Type Conversion{1..2,5..8,10..11} (8 alike) : DataTypeConversion  OutDataTypeStr=boolean
  Data Type Conversion3 : DataTypeConversion
  Data Type Conversion4 : DataTypeConversion  OutDataTypeStr=int8
  Data Type Conversion9 : DataTypeConversion
  EngineCharge Logic : Stateflow chart  TreatAsAtomicUnit=on
  Hood Status : Constant  Value=0
  Rate Transition3 : RateTransition
  RegTrqLimit : Subsystem
  Select_APP : Subsystem
  Sport Mode Enable : Subsystem
  Subsystem1 : Subsystem
  Supervisory  Control  Logic : Stateflow chart  TreatAsAtomicUnit=on
  SysPwrMd : Subsystem
  Terminator1 : Terminator
  Terminator10 : Terminator
  Terminator2 : Terminator
  eSystemStatusVal : Constant  Value=2
  eSystemStatusValidity : Subsystem
  ess.plant.cd_soc_min : Constant  Value=ess.plant.cd_soc_min
  ess.plant.cs_soc_max : Constant  Value=ess.plant.cs_soc_max
  ess.plant.cs_soc_min : Constant  Value=ess.plant.cs_soc_min
  iceSystemStatusVal : Constant  Value=2
  iceSystemStatusValidity : Subsystem
  kph to mph : Gain  Gain=0.6213
  rad/s to RPM : Gain  Gain=30/pi
  Controls : Outport
  tag scope: AccPos_Perc=global, AxlEngTrqCmd=global, AxlMtrTrqCmd=global, BrkMode=global, EnablePrplsn=global, EngAppReq=global, MotorSpeed=global, SportModeEnabled=global, SysPwrMd=global, TransRatio=global, closeMaincReq=global, mode=global, powerMode=global
  wires:
  [BMS_IstSpannung] -> Supervisory  Control  Logic/33(Voltage)
  Bus Selector6/4 -> [BMS_IstSpannung]  "<BMS_IstSpannung>"
  [SW_CS_ON] -> Data Type Conversion11/1
  Data Type Conversion11/1 -> EngineCharge Logic/2(SW_CS_On)
  Data Type Conversion10/1 -> EngineCharge Logic/1(SW_Engine_On)
  [SW_Engine_ON] -> Data Type Conversion10/1
  EngineCharge Logic/1(CDmodeSW) -> Supervisory  Control  Logic/32(CDmode)
  AxlTrq_to_MotTrq/1(Out1) -> RegTrqLimit/1(MotTrqCmd)
  [AxlMtrTrqCmd] -> AxlTrq_to_MotTrq/1(In1)
  [MotorSpeed] -> RegTrqLimit/2(RPM)
  Hood Status/1 -> Supervisory  Control  Logic/31(HoodStatus)
  [plugged] -> Supervisory  Control  Logic/11(plugged)
  AxlTrq_to_EngTrq/1(Out1) -> Bus Creator/10  "EngTrqCmd"
  [closeMaincReq] -> Data Type Conversion/1
  Compare To Constant1/1 -> Bus Creator/1  "SportsModeEnable"
  [EngRunAtv] -> SysPwrMd/2(EngRunAtv)
  [ClutchEngage] -> Bus Creator/18  "ClutchEngage"
  [BPP] -> Bus Creator/19
  [AxlEngTrqCmd] -> AxlTrq_to_EngTrq/1(In1)
  [mode] -> Compare To Constant1/1, Bus Creator/2
  [TransShftLvrPos] -> Bus Creator/13  "TransShftLvrPos"
  [DrvMode] -> Bus Creator/17  "DrvMode"
  [SysPwrMd] -> SysPwrMd/1(SysPwrMd)
  SysPwrMd/1(Out1) -> Bus Creator/12  "SysPwrMd_0_3"
  [VehSpdAvgDrvn] -> Bus Creator/14  "VehSpdAvgDrvn_kph"
  Data Type Conversion9/1 -> Bus Creator/11  "HV_req"
  [BMS_Fehler_Pilot] -> SysPwrMd/4(Fehler_Pilot)
  [EnablePrplsn] -> Bus Creator/5
  [AccPos_Perc] -> 0_to_100/1
  [EnableInverter] -> Bus Creator/9  "EnableInverter"
  [EngOnReq] -> Bus Creator/7  "EngOnReq"
  [HV_req] -> Data Type Conversion9/1
  Select_APP/1(EngAppReq) -> Bus Creator/6  "EngAppReq"
  [BrkMode] -> Bus Creator/16  "BrkMode"
  RegTrqLimit/1(Out1) -> Bus Creator/8  "MtrTrqCmd"
  0_to_100/1 -> Bus Creator/15  "AccPos_Perc"
  [powerMode] -> Bus Creator/3
  Data Type Conversion/1 -> Bus Creator/4  "closeMaincReq"
  [EngOnReq] -> Rate Transition3/1
  Rate Transition3/1 -> SysPwrMd/3(EngOnReq)
  Bus Creator/1 -> Controls/1
  Sensors/1 -> Bus Selector/1, Bus Selector1/1, Bus Selector4/1, Bus Selector6/1, Sport Mode Enable/1(In1)
  Bus Selector/1 -> [TransEstGear]  "<TransEstGear>"
  Bus Selector/2 -> [SysPwrMd]  "<SysPwrMd>"
  Bus Selector/3 -> [BPP]  "<BrkPdlPos>"
  Bus Selector/4 -> [AccPos_Perc]  "<Driver_APP1>"
  Bus Selector/5 -> [VehSpdAvgDrvn]  "<VehSpdAvgDrvn>"
  Bus Selector/6 -> [EngSpd]  "<EngSpd>"
  Bus Selector/7 -> [MotorSpeed]  "<INV_Speed>"
  Bus Selector/9 -> [InverterEnabled]  "<INV_State>"
  Bus Selector1/1 -> [EngRunAtv]  "<EngRunAtv>"
  Bus Selector/8 -> [TransShftLvrPos]  "<TrnsShftLvrPos>"
  Bus Selector1/3 -> [TransRatio]  "<TrnGrRat>"
  Fault Detection/1 -> Bus Selector2/1
  Bus Selector2/1 -> eSystemStatusValidity/1(In1)  "<eSystemStatus>"
  Bus Selector2/2 -> iceSystemStatusValidity/1(In1)  "<iceSystemStatus>"
  Bus Selector4/3 -> Data Type Conversion6/1  "<SW_Regen_Disable>"
  Bus Selector4/1 -> Data Type Conversion7/1  "<SW_CS_ON>"
  Bus Selector4/2 -> Data Type Conversion5/1  "<SW_Engine_ON>"
  eSystemStatusValidity/1(Out1) -> Terminator1/1
  iceSystemStatusValidity/1(Out1) -> Terminator2/1
  Bus Selector/10 -> [plugged]  "<NLG5_S_CP_DT>"
  Data Type Conversion5/1 -> [SW_Engine_ON]
  Data Type Conversion6/1 -> [SW_Regen_Disable]
  Bus Selector6/1 -> [EngFdbkTrq]  "<EngActStdyStTorq>"
  Bus Selector6/2 -> [BMS_Fehler_Pilot]  "<BMS_Fehler_Pilot>"
  Bus Selector6/3 -> [EngCltTmp]  "<EngCltTmp>"
  Bus Selector7/2 -> [FullDrvIntndAxlTrq]  "<FullDrvIntndAxlTrq>"
  Sport Mode Enable/1(Out1) -> [SportModeEnabled]
  Bus Selector1/2 -> [SOC]  "<BMS_SOC>"
  Data Type Conversion7/1 -> [SW_CS_ON]
  Driver Request/1 -> Bus Selector7/1
  Bus Selector7/1 -> [DrvIntndAxlTrq]  "<DrvIntndAxlTrq>"
  Supervisory  Control  Logic/14(ClutchEngage) -> [ClutchEngage]  "ClutchEngage"
  Supervisory  Control  Logic/13(Drvmode) -> [DrvMode]  "DrvMode"
  Supervisory  Control  Logic/10(HV_Req) -> [HV_req]  "HV_req"
  Supervisory  Control  Logic/9(EngTrq) -> [AxlEngTrqCmd]  "EngTrqCmd"
  Supervisory  Control  Logic/7(MotTrqReq) -> [AxlMtrTrqCmd]  "MtrTrqCmd"
  Supervisory  Control  Logic/6(EngOnReq) -> [EngOnReq]  "EngOnReq"
  [SW_CS_ON] -> Subsystem1/2(CS_On)
  [SW_Regen_Disable] -> Supervisory  Control  Logic/23(RegenBrkDisable)
  [SW_CS_ON] -> Supervisory  Control  Logic/21(SW_CS_ON)
  [SportModeEnabled] -> Supervisory  Control  Logic/1(SportModeEnabled)
  Data Type Conversion4/1 -> Supervisory  Control  Logic/3(KeyPos)
  [SysPwrMd] -> Data Type Conversion4/1
  [TransEstGear] -> Supervisory  Control  Logic/2(TransEstGear)
  [BPP] -> Supervisory  Control  Logic/4(BrkPdlPos)
  [AccPos_Perc] -> Supervisory  Control  Logic/5(drvAPP)
  [VehSpdAvgDrvn] -> kph to mph/1
  [EngSpd] -> Supervisory  Control  Logic/7(EngSpd)
  [MotorSpeed] -> rad/s to RPM/1
  [TransShftLvrPos] -> Data Type Conversion3/1
  [InverterEnabled] -> Supervisory  Control  Logic/10(InverterEnabled)
  [SOC] -> Subsystem1/1(SoC)
  [SOC] -> Supervisory  Control  Logic/16(SoC)
  [TransRatio] -> Supervisory  Control  Logic/20(TransRatio)
  [EngRunAtv] -> Supervisory  Control  Logic/15(EngRunAtv)
  [EngFdbkTrq] -> Supervisory  Control  Logic/28(EngFdbkTrq)
  [EngCltTmp] -> Supervisory  Control  Logic/29(EngCtlTmp)
  rad/s to RPM/1 -> Supervisory  Control  Logic/8(MotSpd)
  Supervisory  Control  Logic/5(EngAppReq) -> [EngAppReq]  "EngAppReq"
  eSystemStatusVal/1 -> Supervisory  Control  Logic/24(eSystemStatus)
  iceSystemStatusVal/1 -> Supervisory  Control  Logic/25(iceSystemStatus)
  Data Type Conversion8/1 -> Supervisory  Control  Logic/27(Regen_fault)
  Supervisory  Control  Logic/12(Brkmode) -> [BrkMode]  "BrkMode"
  Subsystem1/1(Faked_SoC) -> Supervisory  Control  Logic/19(Faked_SoC)
  Data Type Conversion1/1 -> Supervisory  Control  Logic/26(ABSAtv)
  Constant3/1 -> Data Type Conversion1/1
  [FullDrvIntndAxlTrq] -> Supervisory  Control  Logic/18(IntdAxleTrq)
  [DrvIntndAxlTrq] -> Supervisory  Control  Logic/17(DrvIntdAxleTrq)
  Supervisory  Control  Logic/11(Chg) -> Terminator10/1
  Constant2/1 -> Data Type Conversion8/1
  kph to mph/1 -> Supervisory  Control  Logic/6(VehicleSpeed)
  Data Type Conversion3/1 -> Supervisory  Control  Logic/9(ShftLvrPos)  "ShftLvrPos"
  Supervisory  Control  Logic/1(mode) -> [mode]  "mode"
  Supervisory  Control  Logic/2(powerMode) -> [powerMode]  "powerMode"
  Supervisory  Control  Logic/3(closeMaincReq) -> [closeMaincReq]  "closeMaincReq"
  Supervisory  Control  Logic/4(EnablePrplsn) -> [EnablePrplsn]  "EnablePrplsn"
  Supervisory  Control  Logic/8(EnableInverter) -> [EnableInverter]  "EnableInverter"
  ess.plant.cs_soc_max/1 -> Supervisory  Control  Logic/14(CS_SOC_MAX)
  ess.plant.cs_soc_min/1 -> Supervisory  Control  Logic/13(CS_SOC_MIN)
  ess.plant.cd_soc_min/1 -> Supervisory  Control  Logic/12(CD_SOC_MIN)
  [SW_Engine_ON] -> Data Type Conversion2/1
  Data Type Conversion2/1 -> Supervisory  Control  Logic/22(SW_Engine_ON)
  [InverterEnabled] -> Supervisory  Control  Logic/30(INV_State)

== system Clutchless_P2_Parallel_ETE/Sensors/CAN/EBCAN/BMS_Antrieb ==
  In1 : Inport
  Bus Creator : BusCreator  Inputs=2
  Bus Selector : BusSelector  OutputSignals=NMH_BMS,ISO_Hybrid_01_Resp
  ISO_Hybrid_01_Resp : Subsystem
  NMH_BMS : Subsystem
  Out1 : Outport
  wires:
  Bus Selector/2 -> ISO_Hybrid_01_Resp/1(In1)  "<ISO_Hybrid_01_Resp>"
  Bus Creator/1 -> Out1/1
  ISO_Hybrid_01_Resp/1(Out1) -> Bus Creator/2
  NMH_BMS/1(Out1) -> Bus Creator/1
  Bus Selector/1 -> NMH_BMS/1(In1)  "<NMH_BMS>"
  In1/1 -> Bus Selector/1

== system Clutchless_P2_Parallel_ETE/Sensors/CAN/EBCAN/CCM ==
  In1 : Inport
  Bus Creator : BusCreator  Inputs=2
  Bus Selector : BusSelector  OutputSignals=NMH_BMS,ISO_Hybrid_01_Resp
  ISO_Hybrid_01_Resp : Subsystem
  NMH_BMS : Subsystem
  Out1 : Outport
  wires:
  In1/1 -> Bus Selector/1
  Bus Selector/1 -> NMH_BMS/1(In1)  "<NMH_BMS>"
  NMH_BMS/1(Out1) -> Bus Creator/1
  ISO_Hybrid_01_Resp/1(Out1) -> Bus Creator/2
  Bus Creator/1 -> Out1/1
  Bus Selector/2 -> ISO_Hybrid_01_Resp/1(In1)  "<ISO_Hybrid_01_Resp>"

== system Clutchless_P2_Parallel_ETE/Sensors/CAN/EBCAN/ECM ==
  In1 : Inport
  Bus Creator : BusCreator  Inputs=7
  Bus Selector : BusSelector  OutputSignals=Sensors_to_ECM.EngActStdyStTorq_Nm,Sensors_to_ECM.EngSpd_RPM,ECM_to_Actuators.VehSpdAvgDrvn,ECM_to_Actuators.EngRunAtv,ECM_to_Actuators.Eng_Temp,ECM_to_Actuators.ECM_RollingAliveCnt
  Data Type Conversion{1..6} (6 alike) : DataTypeConversion
  ETEI_Engine_Torque_Status : Subsystem
  Ground : Ground
  PPEI_Engine_General_Status_4 : Subsystem
  PPEI_Engine_General_Status_6 : Subsystem
  PPEI_Vehicle_Speed_and_Distance : Subsystem
  PTEI_Engine_Torque_Status : Subsystem
  Out1 : Outport
  wires:
  Data Type Conversion1/1 -> Bus Creator/4  "EngRunAtv"
  Data Type Conversion3/1 -> Bus Creator/2  "EngSpd"
  PPEI_Engine_General_Status_6/1(Out1) -> Bus Creator/7
  Data Type Conversion6/1 -> PPEI_Engine_General_Status_6/1(In1)
  PPEI_Engine_General_Status_4/1(Out1) -> Bus Creator/6
  Data Type Conversion5/1 -> PPEI_Engine_General_Status_4/1(In1)
  PTEI_Engine_Torque_Status/1(Out1) -> Bus Creator/5
  Ground/1 -> PTEI_Engine_Torque_Status/1(In1)
  Bus Selector/4 -> Data Type Conversion1/1  "<EngRunAtv>"
  Bus Creator/1 -> Out1/1
  PPEI_Vehicle_Speed_and_Distance/1(Out1) -> Bus Creator/3
  ETEI_Engine_Torque_Status/1(Out1) -> Bus Creator/1
  Data Type Conversion4/1 -> PPEI_Vehicle_Speed_and_Distance/1(In1)
  Bus Selector/2 -> Data Type Conversion3/1  "<EngSpd_RPM>"
  Data Type Conversion2/1 -> ETEI_Engine_Torque_Status/1(In1)
  In1/1 -> Bus Selector/1
  Bus Selector/1 -> Data Type Conversion2/1  "<EngActStdyStTorq_Nm>"
  Bus Selector/3 -> Data Type Conversion4/1  "<VehSpdAvgDrvn>"
  Bus Selector/5 -> Data Type Conversion5/1  "<Eng_Temp>"
  Bus Selector/6 -> Data Type Conversion6/1  "<ECM_RollingAliveCnt>"

== system Clutchless_P2_Parallel_ETE/Sensors/CAN/HV_CAN/BMS_Hybrid ==
  In1 : Inport
  BMS_HYB_02 : Subsystem
  BMS_HYB_03 : Subsystem
  BMS_HYB_04 : Subsystem
  Bus Creator : BusCreator  Inputs=6
  Bus Selector : BusSelector  OutputSignals=BMS_HYB_02,BMS_HYB_04,BMS_HYB_03,BMS_HYB_02.BMS_Fehler_Isolation,BMS_HYB_06.BMS_Temperatur,BMS_HYB_02.BMS_Fehler_HS_verschweisst
  Data Type Conversion : DataTypeConversion
  Data Type Conversion1 : DataTypeConversion
  Data Type Conversion2 : DataTypeConversion
  Out1 : Outport
  wires:
  Data Type Conversion2/1 -> Bus Creator/6  "BMS_Fehler_HS_verschweisst"
  Bus Selector/5 -> Data Type Conversion/1  "<BMS_Temperatur>"
  Bus Selector/4 -> Data Type Conversion1/1  "<BMS_Fehler_Isolation>"
  BMS_HYB_03/1(Out1) -> Bus Creator/3
  Bus Selector/3 -> BMS_HYB_03/1(In1)  "<BMS_HYB_03>"
  BMS_HYB_04/1(Out1) -> Bus Creator/2
  BMS_HYB_02/1(Out1) -> Bus Creator/1
  Bus Creator/1 -> Out1/1
  Bus Selector/2 -> BMS_HYB_04/1(In1)  "<BMS_HYB_04>"
  Bus Selector/1 -> BMS_HYB_02/1(In1)  "<BMS_HYB_02>"
  In1/1 -> Bus Selector/1
  Data Type Conversion/1 -> Bus Creator/5  "BMS_Temperatur"
  Data Type Conversion1/1 -> Bus Creator/4  "BMS_Fehler_Isolation"
  Bus Selector/6 -> Data Type Conversion2/1  "<BMS_Fehler_HS_verschweisst>"

== system Clutchless_P2_Parallel_ETE/Sensors/CAN/HV_CAN/MCU ==
  In1 : Inport
  Bus Creator : BusCreator  Inputs=6
  Bus Creator1 : BusCreator  Inputs=2
  Bus Creator2 : BusCreator  Inputs=2
  Bus Selector : BusSelector  OutputSignals=Sensors_to_MCU.mot_spd_out,Sensors_to_MCU.mot_crr_out,MCU_to _Actuator.InverterEnabled,MCU_to _Actuator.MotTrqFdbck,MCU_to _Actuator.D3_Power_On_Timer,Sensors_to_MCU.mot_volt_in
  Bus Selector1 : BusSelector  OutputSignals=Sensors_to_MCU.mcu_temp,Sensors_to_MCU.mot_temp
  Data Type Conversion{1..5,7..9} (8 alike) : DataTypeConversion
  In2 : InportShadow
  Out1 : Outport
  wires:
  In1/1 -> Bus Selector/1
  Bus Selector/6 -> Data Type Conversion9/1  "<mot_volt_in>"
  Bus Selector/4 -> Data Type Conversion7/1  "<MotTrqFdbck>"
  Bus Selector/5 -> Data Type Conversion8/1  "<D3_Power_On_Timer>"
  Bus Creator/1 -> Bus Creator1/1  "INV_VCU_01"
  Data Type Conversion3/1 -> Bus Creator/3  "INV_State"
  Data Type Conversion2/1 -> Bus Creator/2  "INV_CurrentHV"
  Data Type Conversion1/1 -> Bus Creator/1  "INV_Speed"
  Bus Selector/3 -> Data Type Conversion3/1  "<InverterEnabled>"
  Bus Selector/2 -> Data Type Conversion2/1  "<mot_crr_out>"
  Bus Selector/1 -> Data Type Conversion1/1  "<mot_spd_out>"
  Data Type Conversion7/1 -> Bus Creator/4  "INV_OutputTorque"
  Data Type Conversion8/1 -> Bus Creator/5  "MessageCounter_200"
  Data Type Conversion9/1 -> Bus Creator/6  "INV_VoltageHV"
  Data Type Conversion4/1 -> Bus Creator2/1  "INV_InverterTemperature"
  Bus Selector1/2 -> Data Type Conversion5/1  "<mot_temp>"
  Data Type Conversion5/1 -> Bus Creator2/2  "INV_ElectricMachineTemperature"
  Bus Selector1/1 -> Data Type Conversion4/1  "<mcu_temp>"
  In2/1 -> Bus Selector1/1
  Bus Creator2/1 -> Bus Creator1/2  "INV_VCU_04"
  Bus Creator1/1 -> Out1/1

== system Clutchless_P2_Parallel_ETE/Sensors/CAN/HV_CAN/OBC ==
  In1 : Inport
  Bus Creator : BusCreator  Inputs=5
  Bus Selector : BusSelector  OutputSignals=NLG5_ACT_I,NLG5_ACT_II,NLG5_ERR,NLG5_ST,NLG5_TEMP
  NLG5_ACT_I : Subsystem
  NLG5_ACT_II : Subsystem
  NLG5_ERR : Subsystem
  NLG5_ST : Subsystem
  NLG5_TEMP : Subsystem
  Out1 : Outport
  wires:
  In1/1 -> Bus Selector/1
  Bus Selector/1 -> NLG5_ACT_I/1(In1)  "<NLG5_ACT_I>"
  NLG5_ACT_I/1(Out1) -> Bus Creator/1
  Bus Selector/2 -> NLG5_ACT_II/1(In1)  "<NLG5_ACT_II>"
  NLG5_ACT_II/1(Out1) -> Bus Creator/2
  NLG5_ERR/1(Out1) -> Bus Creator/3
  Bus Selector/3 -> NLG5_ERR/1(In1)  "<NLG5_ERR>"
  Bus Selector/4 -> NLG5_ST/1(In1)  "<NLG5_ST>"
  NLG5_ST/1(Out1) -> Bus Creator/4
  Bus Selector/5 -> NLG5_TEMP/1(In1)  "<NLG5_TEMP>"
  NLG5_TEMP/1(Out1) -> Bus Creator/5
  Bus Creator/1 -> Out1/1

== system Clutchless_P2_Parallel_ETE/Sensors/CAN/VEH_CAN/BCM ==
  In1 : Inport
  Bus Creator : BusCreator  Inputs=2
  Bus Selector : BusSelector  OutputSignals=SysPwrMd,BrkPdlPos
  Data Type Conversion : DataTypeConversion
  Data Type Conversion1 : DataTypeConversion
  PPEI_Brake_Apply_Status : Subsystem
  PPEI_Platfrom_General_Status : Subsystem
  Out1 : Outport
  wires:
  Data Type Conversion1/1 -> PPEI_Brake_Apply_Status/1(In1)
  Data Type Conversion/1 -> PPEI_Platfrom_General_Status/1(In1)
  Bus Creator/1 -> Out1/1
  PPEI_Brake_Apply_Status/1(Out1) -> Bus Creator/2
  PPEI_Platfrom_General_Status/1(Out1) -> Bus Creator/1
  Bus Selector/2 -> Data Type Conversion1/1  "<BrkPdlPos>"
  Bus Selector/1 -> Data Type Conversion/1  "<SysPwrMd>"
  In1/1 -> Bus Selector/1

== system Clutchless_P2_Parallel_ETE/Sensors/CAN/VEH_CAN/EBCM ==
  In1 : Inport
  Bus Selector : BusSelector  OutputSignals=PPEI_Chassis_General_Status_1.BrkPdlDrvAppPrsDetcd
  Constant : Constant  OutDataTypeStr=boolean
  PPEI_Chassis_General_Status_1 : Subsystem
  Terminator : Terminator
  Out1 : Outport
  wires:
  Constant/1 -> PPEI_Chassis_General_Status_1/1(In1)
  In1/1 -> Bus Selector/1
  PPEI_Chassis_General_Status_1/1(Out1) -> Out1/1
  Bus Selector/1 -> Terminator/1  "<BrkPdlDrvAppPrsDetcd>"

== system Clutchless_P2_Parallel_ETE/Sensors/CAN/VEH_CAN/ICCM ==
  In1 : Inport
  Out1 : Outport
  wires:
  In1/1 -> Out1/1

== system Clutchless_P2_Parallel_ETE/Sensors/CAN/VEH_CAN/TCM ==
  In1 : Inport
  Bus Creator : BusCreator  Inputs=4
  Bus Selector : BusSelector  OutputSignals=TCM_to _Actuator.TransEstGear,TCM_to _Actuator.LockupCmd,TCM_to _Actuator.TrnsShftLvrPos,Sensors_to_TCM.gb_trq_ratio
  Data Type Conversion{,1..3} (4 alike) : DataTypeConversion
  Out1 : Outport
  wires:
  Data Type Conversion/1 -> Bus Creator/1  "TransEstGear"
  Bus Creator/1 -> Out1/1
  In1/1 -> Bus Selector/1
  Data Type Conversion1/1 -> Bus Creator/2  "TrnsTrqCnvCltCmndMd"
  Data Type Conversion2/1 -> Bus Creator/3  "TrnsShftLvrPos"
  Data Type Conversion3/1 -> Bus Creator/4  "TrnGrRat"
  Bus Selector/1 -> Data Type Conversion/1  "<TransEstGear>"
  Bus Selector/2 -> Data Type Conversion1/1  "<LockupCmd>"
  Bus Selector/3 -> Data Type Conversion2/1  "<TrnsShftLvrPos>"
  Bus Selector/4 -> Data Type Conversion3/1  "<gb_trq_ratio>"

== system Clutchless_P2_Parallel_ETE/Camaro Plant Model/E-Machine/IMG Plant/Electric Machine/Calculate Mot Efficiency, MotPwrMech, and, MotPwrElec1 ==
  note: Pelec_req = Pmech_req*Eff^k,
      | k = -1 if Trq >= 0,
      | k = 1 if Trq < 0
  MotSpd : Inport
  MotTrqAct : Inport  Port=2
  -1 : Gain  Gain=8
  "-1 when + 1 when - " : Gain  Gain=-1
  -2 : Gain  Gain=tloop
  2-D Lookup Table : Lookup_n-D  BreakpointsForDimension1=mot.plant.init.eff_trq.idx2_trq  BreakpointsForDimension2=mot.plant.init.eff_trq.idx1_spd  Table=mot.plant.init.eff_trq.map  InternalRulePriority=Speed  RndMeth=Simplest  InputSameDT=on
  Abs{,1..3} (4 alike) : Abs
  Add : Sum  Inputs=-+
  Add1 : Sum  Inputs=+-
  Constant : Constant  Value=1-0.8
  Gain2 : Gain  Gain=1/100
  MCU_WEGPmp : Constant  Value=0
  Math Function1 : Math  Operator=pow  SaturateOnIntegerOverflow=on
  Memory : Memory
  Product : Product
  Product1 : Product
  Product2 : Product
  Sign : Signum
  rad/s to rpm : Gain  Gain=30/pi
  Losses : Outport
  MCU_Heat : Outport  Port=2
  MotPwrElec : Outport  Port=3
  wires:
  -2/1 -> MCU_Heat/1
  -1/1 -> Add1/2
  Add1/1 -> -2/1
  MCU_WEGPmp/1 -> -1/1
  Abs3/1 -> Add1/1
  Product2/1 -> Abs3/1
  Constant/1 -> Product2/2
  Memory/1 -> Sign/1
  Math Function1/1 -> Product1/2
  Add/1 -> Abs2/1
  Abs2/1 -> Losses/1
  "-1 when + 1 when - "/1 -> Math Function1/2
  MotSpd/1 -> rad/s to rpm/1, Product/2
  MotTrqAct/1 -> Abs/1, Product/1, Memory/1
  Product/1 -> Product1/1, Add/1  "MotPwrMech"
  Product1/1 -> Add/2, Product2/1, MotPwrElec/1  "MotPwrElec"
  2-D Lookup Table/1 -> Gain2/1
  Gain2/1 -> Math Function1/1
  Abs/1 -> 2-D Lookup Table/1
  Sign/1 -> "-1 when + 1 when - "/1
  Abs1/1 -> 2-D Lookup Table/2
  rad/s to rpm/1 -> Abs1/1

== system Clutchless_P2_Parallel_ETE/Camaro Plant Model/E-Machine/IMG Plant/Electric Machine/MotTrqExcessTrigger1 ==
  In1 : Inport
  Bias : Bias  Bias=55
  Bias1 : Bias  Bias=25
  Constant : Constant  Value=0
  Multiport Switch : MultiPortSwitch  DataPortOrder=Zero-based contiguous
  Terminator : Terminator
  Out1 : Outport
  tag scope: MotTrqExcessTrig=global
  wires:
  Constant/1 -> Multiport Switch/1, [MotTrqExcessTrig]
  Bias1/1 -> Multiport Switch/3
  In1/1 -> Bias1/1, Bias/1, Multiport Switch/2
  Bias/1 -> Multiport Switch/4
  Multiport Switch/1 -> Out1/1
  [MotTrqExcessTrig] -> Terminator/1

== system Clutchless_P2_Parallel_ETE/Camaro Plant Model/E-Machine/IMG Plant/Electric Machine/Thermal1 ==
  Losses : Inport
  MCU_heat : Inport  Port=2
  MotInv_loop : Subsystem
  Motor Thermal : Subsystem  Commented=on
  MCU_temp_C : Outport
  motor_temp : Outport  Port=2
  wires:
  MotInv_loop/2(Out2) -> motor_temp/1
  MotInv_loop/1(Out1) -> MCU_temp_C/1
  Losses/1 -> MotInv_loop/1(In1)  "[W]"
  MCU_heat/1 -> MotInv_loop/2(In2)

== system Clutchless_P2_Parallel_ETE/Camaro Plant Model/E-Machine/IMG Plant/Electric Machine/Torque Calculation1 ==
  MotSpd : Inport
  MotTrqCmd : Inport  Port=2
  Abs : Abs
  Abs1 : Abs
  Memory : Memory
  MinMax : MinMax  Inputs=2
  Product : Product
  Sign : Signum
  electric machine filter : Subsystem
  "max torque " : Subsystem
  mot_trq_out : Outport
  wires:
  Product/1 -> Memory/1
  MotTrqCmd/1 -> Abs/1, Sign/1, "max torque "/1(cmd)
  electric machine filter/1(filtered) -> mot_trq_out/1
  Abs1/1 -> MinMax/2
  Abs/1 -> MinMax/1
  MinMax/1 -> Product/2
  Sign/1 -> Product/1
  MotSpd/1 -> "max torque "/2(speed)
  "max torque "/1(max torque) -> Abs1/1
  Memory/1 -> electric machine filter/1(trq)

== system Clutchless_P2_Parallel_ETE/Camaro Plant Model/E-Machine/IMG Plant/Electric Machine/non-zero division1 ==
  note: and finally, the expression is: (u[1] \ u[2]) * 1 = u[1] \ u[2]
  note: (u[2]!=0) is true then returns 1
  note: if u[2] != 0, then output == u[1]\u[2]:
  note: (u[2]==0) is false then returns 0, thus (u[2]+(u[2]==0)) is equal to u[2]+0=u[2]
  note: and finally, the expression is: (u[1] \ 1) * 0 = 0
  note: (u[2]!=0) is false then returns 0
  note: if u[2] == 0, then output == 0:
  note: (u[2]==0) is true then returns 1, thus (u[2]+(u[2]==0)) is equal to 0+1=1
  note: original idea from Phil Sharer - ANL
      | original formula: u[1]\(u[2]+eps)*(u[2]!=0)
      | changes done by Gerald ZINI (dgey) - ANL (05\02\2001)
  In1 : Inport
  In2 : Inport  Port=2
  Fcn : Fcn  Expr=u[1]/(u[2]+(u[2]==0))*(u[2]!=0)
  Mux : Mux  Inputs=2
  Out1 : Outport
  wires:
  In2/1 -> Mux/2
  Fcn/1 -> Out1/1
  In1/1 -> Mux/1
  Mux/1 -> Fcn/1

== system Clutchless_P2_Parallel_ETE/Camaro Plant Model/E-Machine/IMG Plant2/Calculate Mot Efficiency, MotPwrMech, and, MotPwrElec/Lower Limit ==
  In1 : Inport
  Constant3 : Constant  Value=Lolimit
  MinMax : MinMax  Function=max  Inputs=2
  Out1 : Outport
  wires:
  MinMax/1 -> Out1/1
  Constant3/1 -> MinMax/2
  In1/1 -> MinMax/1

== system Clutchless_P2_Parallel_ETE/Camaro Plant Model/E-Machine/IMG Plant2/Calculate Mot Efficiency, MotPwrMech, and, MotPwrElec/MCUOverTemp Fault ==
  In1 : Inport
  Gain : Gain  Gain=3
  Switch : Switch  Threshold=1
  Out1 : Outport
  wires:
  Switch/1 -> Out1/1
  Gain/1 -> Switch/1
  [MCUOverTemp] -> Switch/2
  In1/1 -> Gain/1, Switch/3
